simulink model "DC_Motor_project_TET4120 (1)"  (R2024b)
settings: Solver=ode23tb  StartTime=0.0  StopTime=1.2  MaxStep=10e-6  RelTol=1e-3  EnableMultiTasking=on
values from neighbouring files (symbols this model uses):
  A = 2.5    [Other_model_parameters.m]
  c_w = 0.2    [Other_model_parameters.m]
  g = 9.81    [Other_model_parameters.m]
  i_g = 10    [Other_model_parameters.m]
  J = J_car + J_m + J_g    (= 0.50375)    [Other_model_parameters.m]
  M = 2200    [Other_model_parameters.m]
  mu_r = 0.01    [Other_model_parameters.m]
  r_w = 0.25    [Other_model_parameters.m]
  rho = 1.2    [Other_model_parameters.m]
undefined symbols (not defined in the file or in its folder): DiscIntNeverNeededParam, eea_lib, PI, reg
libraries: spsVoltageMeasurementLib x8, simulink_extras x6, spsCurrentMeasurementLib x4, spsOnDelayLib x2, spsMonostableLib x2, spsControlledCurrentSourceLib x2, spsUniversalBridgeLib x2, spsDCVoltageSourceLib x1, sps_lib x1
(part 2 of 2)

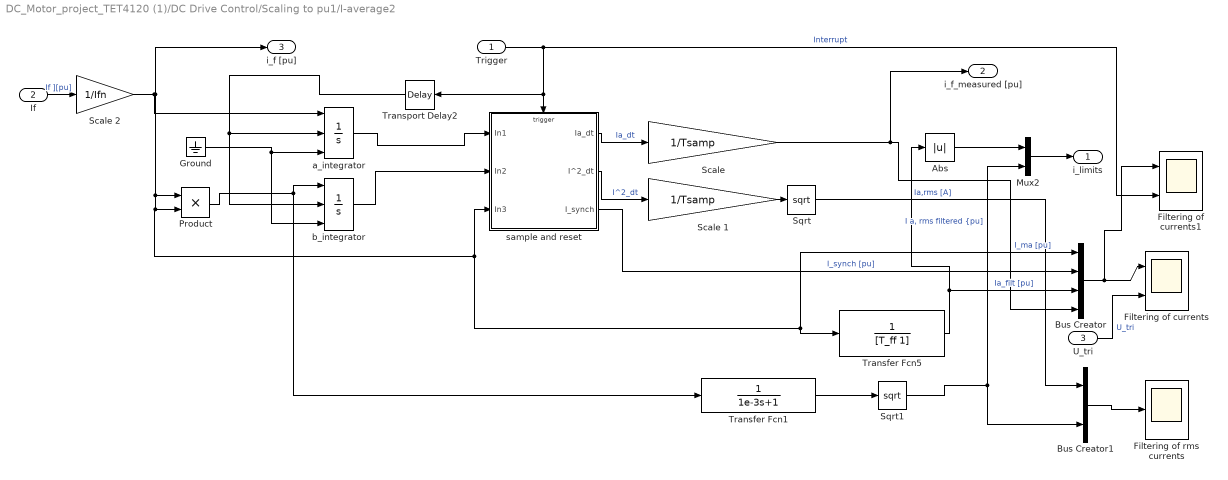
== system DC_Motor_project_TET4120 (1)/DC Drive Control/Scaling to pu1/I-average2 ==
  Trigger : Inport
  If : Inport  Port=2
  U_tri : Inport  Port=3
  Abs : Abs  SaturateOnIntegerOverflow=off
  Bus Creator : BusCreator  Inputs=4
  Bus Creator1 : BusCreator  Inputs=2
  Filtering of currents : Scope  NumInputPorts=2
  Filtering of currents1 : Scope  NumInputPorts=2
  Filtering of rms currents : Scope
  Ground : Ground
  Mux2 : Mux  Inputs=2
  Product : Product  RndMeth=Zero
  "Scale " : Gain  Gain=1/Tsamp
  Scale 1 : Gain  Gain=1/Tsamp
  Scale 2 : Gain  Gain=1/Ifn
  Sqrt : Sqrt
  Sqrt1 : Sqrt
  Transfer Fcn1 : TransferFcn  Denominator=[1e-3 1]
  Transfer Fcn5 : TransferFcn  Denominator=[T_ff 1]
  Transport Delay2 : TransportDelay  DelayTime=1e-12
  a_integrator : Integrator  ExternalReset=rising  InitialConditionSource=external
  b_integrator : Integrator  ExternalReset=rising  InitialConditionSource=external
  sample and reset : Subsystem
  i_limits : Outport
  i_f_measured [pu] : Outport  Port=2
  i_f [pu] : Outport  Port=3
  wires:
  Sqrt/1 -> Bus Creator1/1  "Ia,rms [A]"
  Scale 1/1 -> Sqrt/1
  sample and reset/2(I^2_dt) -> Scale 1/1  "I^2_dt"
  "Scale "/1 -> i_f_measured [pu]/1, Bus Creator/4  "I_ma [pu]"
  sample and reset/1(Ia_dt) -> "Scale "/1  "Ia_dt"
  Product/1 -> b_integrator/1, Transfer Fcn1/1
  Mux2/1 -> i_limits/1
  Transport Delay2/1 -> b_integrator/2, a_integrator/2
  Ground/1 -> b_integrator/3, a_integrator/3
  a_integrator/1 -> sample and reset/1(In1)
  Trigger/1 -> Filtering of currents1/2, Transport Delay2/1, sample and reset/Trigger  "Interrupt"
  Transfer Fcn5/1 -> Bus Creator/3, Abs/1  "Ia_filt [pu]"
  Transfer Fcn1/1 -> Sqrt1/1
  Abs/1 -> Mux2/1
  If/1 -> Scale 2/1  "If ][pu]"
  b_integrator/1 -> sample and reset/2(In2)
  sample and reset/3(I_synch) -> Bus Creator/2  "I_synch [pu]"
  Sqrt1/1 -> Bus Creator1/2, Mux2/2  "I a, rms filtered {pu]"
  Bus Creator/1 -> Filtering of currents1/1, Filtering of currents/1
  Bus Creator1/1 -> Filtering of rms currents/1
  U_tri/1 -> Filtering of currents/2  "U_tri"
  Scale 2/1 -> Bus Creator/1, Transfer Fcn5/1, sample and reset/3(In3), Product/2, Product/1, i_f [pu]/1, a_integrator/1

== system DC_Motor_project_TET4120 (1)/DC Drive Control/Speed Controller/Speed controller  ==
  e : Inport
  UL : Inport  Port=2
  LL : Inport  Port=3
  Abs : Abs  SaturateOnIntegerOverflow=off
  Integral : UnitDelay  SampleTime=-1  HasFrameUpgradeWarning=on
  Kp : Gain  Gain=Kp  SaturateOnIntegerOverflow=on  OutDataTypeStr=Inherit: Same as input  ParamDataTypeStr=Inherit: Same as input
  Lim1 : Subsystem
      mask Display:
      | plot([0.3 0.5 0.7 0.3], [0.1 0.3  0.1 0.1])
      | plot([0.3 0.5 0.7 0.3], [0.9 0.7  0.9 0.9])
  Sum1 : Sum  Inputs=|+-  InputSameDT=on  SaturateOnIntegerOverflow=on  OutDataTypeStr=Inherit: Same as first input
  Sum4 : Sum  Inputs=++|  InputSameDT=on  SaturateOnIntegerOverflow=on  OutDataTypeStr=Inherit: Same as first input
  Switch4 : Switch  Threshold=0.5
  in Limit : Relay  OffSwitchValue=0
  Out : Outport
  wires:
  e/1 -> Kp/1  "e"
  Kp/1 -> Sum4/2
  UL/1 -> Lim1/1(UL)
  Lim1/1(Out) -> Sum1/1, Out/1
  Integral/1 -> Sum4/1, Switch4/1  "intergral"
  Sum4/1 -> Sum1/2, Lim1/2(In), Switch4/3  "u_r"
  LL/1 -> Lim1/3(LL)
  Abs/1 -> in Limit/1
  Sum1/1 -> Abs/1
  in Limit/1 -> Switch4/2  "saturation"
  Switch4/1 -> Integral/1

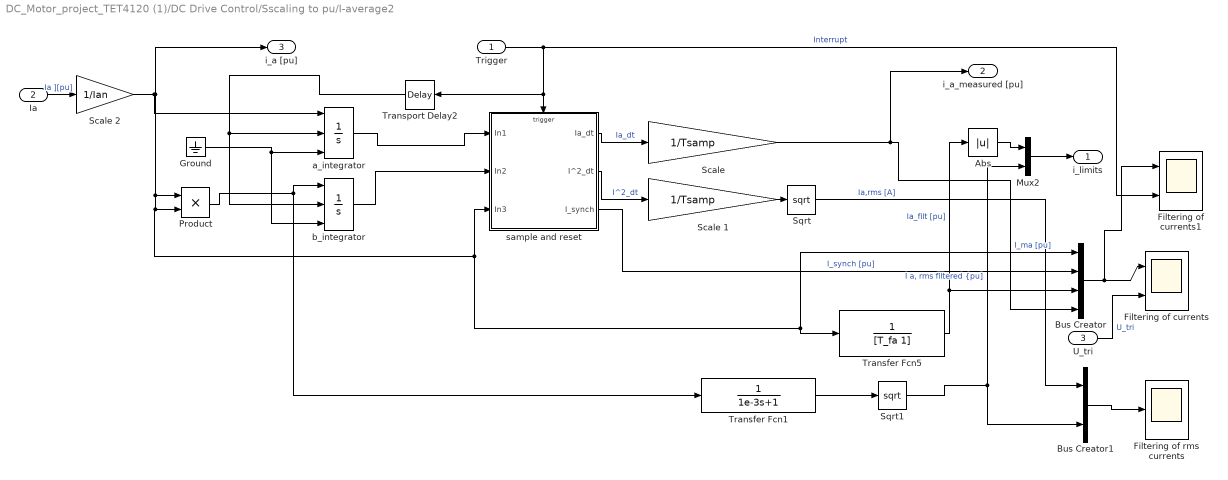
== system DC_Motor_project_TET4120 (1)/DC Drive Control/Sscaling to pu/I-average2 ==
  Trigger : Inport
  Ia : Inport  Port=2
  U_tri : Inport  Port=3
  Abs : Abs  SaturateOnIntegerOverflow=off
  Bus Creator : BusCreator  Inputs=4
  Bus Creator1 : BusCreator  Inputs=2
  Filtering of currents : Scope  NumInputPorts=2
  Filtering of currents1 : Scope  NumInputPorts=2
  Filtering of rms currents : Scope
  Ground : Ground
  Mux2 : Mux  Inputs=2
  Product : Product  RndMeth=Zero
  "Scale " : Gain  Gain=1/Tsamp
  Scale 1 : Gain  Gain=1/Tsamp
  Scale 2 : Gain  Gain=1/Ian
  Sqrt : Sqrt
  Sqrt1 : Sqrt
  Transfer Fcn1 : TransferFcn  Denominator=[1e-3 1]
  Transfer Fcn5 : TransferFcn  Denominator=[T_fa 1]
  Transport Delay2 : TransportDelay  DelayTime=1e-12
  a_integrator : Integrator  ExternalReset=rising  InitialConditionSource=external
  b_integrator : Integrator  ExternalReset=rising  InitialConditionSource=external
  sample and reset : Subsystem
  i_limits : Outport
  i_a_measured [pu] : Outport  Port=2
  i_a [pu] : Outport  Port=3
  wires:
  Sqrt/1 -> Bus Creator1/1  "Ia,rms [A]"
  Scale 1/1 -> Sqrt/1
  sample and reset/2(I^2_dt) -> Scale 1/1  "I^2_dt"
  "Scale "/1 -> i_a_measured [pu]/1, Bus Creator/4  "I_ma [pu]"
  sample and reset/1(Ia_dt) -> "Scale "/1  "Ia_dt"
  Product/1 -> b_integrator/1, Transfer Fcn1/1
  Mux2/1 -> i_limits/1
  Transport Delay2/1 -> b_integrator/2, a_integrator/2
  Ground/1 -> b_integrator/3, a_integrator/3
  a_integrator/1 -> sample and reset/1(In1)
  Trigger/1 -> Filtering of currents1/2, Transport Delay2/1, sample and reset/Trigger  "Interrupt"
  Transfer Fcn5/1 -> Bus Creator/3, Abs/1  "Ia_filt [pu]"
  Transfer Fcn1/1 -> Sqrt1/1
  Abs/1 -> Mux2/1
  Ia/1 -> Scale 2/1  "Ia ][pu]"
  b_integrator/1 -> sample and reset/2(In2)
  sample and reset/3(I_synch) -> Bus Creator/2  "I_synch [pu]"
  Sqrt1/1 -> Bus Creator1/2, Mux2/2  "I a, rms filtered {pu]"
  Bus Creator/1 -> Filtering of currents1/1, Filtering of currents/1
  Bus Creator1/1 -> Filtering of rms currents/1
  U_tri/1 -> Filtering of currents/2  "U_tri"
  Scale 2/1 -> Bus Creator/1, Transfer Fcn5/1, sample and reset/3(In3), Product/2, Product/1, i_a [pu]/1, a_integrator/1

== system DC_Motor_project_TET4120 (1)/DC Drive Control/pwm modulator1/Subsystem ==
  time : Inport
  T_tri : Inport  Port=2
  Abs : Abs
  Bus Creator : BusCreator  Inputs=2
  Constant1 : Constant  Value=4
  Constant2 : Constant
  Gain : Gain  Gain=-1  SaturateOnIntegerOverflow=on  OutDataTypeStr=Inherit: Same as input  ParamDataTypeStr=Inherit: Same as input
  Gain1 : Gain  Gain=-1  SaturateOnIntegerOverflow=on  OutDataTypeStr=Inherit: Same as input  ParamDataTypeStr=Inherit: Same as input
  Product : Product  InputSameDT=on  SaturateOnIntegerOverflow=on  OutDataTypeStr=Inherit: Same as first input
  Product1 : Product  Inputs=*/  InputSameDT=on  SaturateOnIntegerOverflow=on  OutDataTypeStr=Inherit: Same as first input
  Product2 : Product  InputSameDT=on  SaturateOnIntegerOverflow=on  OutDataTypeStr=Inherit: Same as first input
  Product3 : Product  Inputs=*/  InputSameDT=on  SaturateOnIntegerOverflow=on  OutDataTypeStr=Inherit: Same as first input
  Rounding Function : Rounding  Operator=round
  Sum : Sum  Inputs=-+  InputSameDT=on  SaturateOnIntegerOverflow=on  OutDataTypeStr=Inherit: Same as first input
  Sum1 : Sum  Inputs=-+  InputSameDT=on  SaturateOnIntegerOverflow=on  OutDataTypeStr=Inherit: Same as first input
  Out1 : Outport
  wires:
  time/1 -> Sum/1, Product1/1
  T_tri/1 -> Product3/2, Product/2, Product1/2
  Product1/1 -> Rounding Function/1
  Rounding Function/1 -> Product/1
  Product/1 -> Sum/2
  Sum/1 -> Product2/1
  Gain/1 -> Product2/2
  Constant1/1 -> Product3/1
  Product3/1 -> Gain/1
  Product2/1 -> Abs/1
  Abs/1 -> Sum1/2
  Constant2/1 -> Sum1/1
  Gain1/1 -> Bus Creator/1
  Sum1/1 -> Gain1/1, Bus Creator/2
  Bus Creator/1 -> Out1/1

== system DC_Motor_project_TET4120 (1)/DC Drive Control/pwm modulator2/Subsystem ==
  time : Inport
  T_tri : Inport  Port=2
  Abs : Abs
  Bus Creator : BusCreator  Inputs=2
  Constant1 : Constant  Value=4
  Constant2 : Constant
  Gain : Gain  Gain=-1  SaturateOnIntegerOverflow=on  OutDataTypeStr=Inherit: Same as input  ParamDataTypeStr=Inherit: Same as input
  Gain1 : Gain  Gain=-1  SaturateOnIntegerOverflow=on  OutDataTypeStr=Inherit: Same as input  ParamDataTypeStr=Inherit: Same as input
  Product : Product  InputSameDT=on  SaturateOnIntegerOverflow=on  OutDataTypeStr=Inherit: Same as first input
  Product1 : Product  Inputs=*/  InputSameDT=on  SaturateOnIntegerOverflow=on  OutDataTypeStr=Inherit: Same as first input
  Product2 : Product  InputSameDT=on  SaturateOnIntegerOverflow=on  OutDataTypeStr=Inherit: Same as first input
  Product3 : Product  Inputs=*/  InputSameDT=on  SaturateOnIntegerOverflow=on  OutDataTypeStr=Inherit: Same as first input
  Rounding Function : Rounding  Operator=round
  Sum : Sum  Inputs=-+  InputSameDT=on  SaturateOnIntegerOverflow=on  OutDataTypeStr=Inherit: Same as first input
  Sum1 : Sum  Inputs=-+  InputSameDT=on  SaturateOnIntegerOverflow=on  OutDataTypeStr=Inherit: Same as first input
  Out1 : Outport
  wires:
  time/1 -> Sum/1, Product1/1
  T_tri/1 -> Product3/2, Product/2, Product1/2
  Product1/1 -> Rounding Function/1
  Rounding Function/1 -> Product/1
  Product/1 -> Sum/2
  Sum/1 -> Product2/1
  Gain/1 -> Product2/2
  Constant1/1 -> Product3/1
  Product3/1 -> Gain/1
  Product2/1 -> Abs/1
  Abs/1 -> Sum1/2
  Constant2/1 -> Sum1/1
  Gain1/1 -> Bus Creator/1
  Sum1/1 -> Gain1/1, Bus Creator/2
  Bus Creator/1 -> Out1/1

== system DC_Motor_project_TET4120 (1)/DC Drive Control/task manager1/Boolean delay ==
  In1 : Inport
  Data Type Conversion1 : DataTypeConversion  OutDataTypeStr=double  SaturateOnIntegerOverflow=off  RndMeth=Floor
  Data Type Conversion2 : DataTypeConversion  OutDataTypeStr=boolean  SaturateOnIntegerOverflow=off  RndMeth=Floor
  Transport Delay4 : TransportDelay  DelayTime=T_exec_0
  Out1 : Outport
  wires:
  Data Type Conversion2/1 -> Out1/1
  In1/1 -> Data Type Conversion1/1
  Transport Delay4/1 -> Data Type Conversion2/1
  Data Type Conversion1/1 -> Transport Delay4/1

== system DC_Motor_project_TET4120 (1)/DC Drive Control/task manager1/Boolean delay1 ==
  In1 : Inport
  Data Type Conversion1 : DataTypeConversion  OutDataTypeStr=double  SaturateOnIntegerOverflow=off  RndMeth=Floor
  Data Type Conversion2 : DataTypeConversion  OutDataTypeStr=boolean  SaturateOnIntegerOverflow=off  RndMeth=Floor
  Transport Delay4 : TransportDelay  DelayTime=T_exec_0
  Out1 : Outport
  wires:
  Data Type Conversion1/1 -> Transport Delay4/1
  Transport Delay4/1 -> Data Type Conversion2/1
  In1/1 -> Data Type Conversion1/1
  Data Type Conversion2/1 -> Out1/1

== system DC_Motor_project_TET4120 (1)/DC Drive Control/task manager1/Boolean delay2 ==
  In1 : Inport
  Data Type Conversion1 : DataTypeConversion  OutDataTypeStr=double  SaturateOnIntegerOverflow=off  RndMeth=Floor
  Data Type Conversion2 : DataTypeConversion  OutDataTypeStr=boolean  SaturateOnIntegerOverflow=off  RndMeth=Floor
  Transport Delay4 : TransportDelay  DelayTime=T_exec_0
  Out1 : Outport
  wires:
  Data Type Conversion2/1 -> Out1/1
  In1/1 -> Data Type Conversion1/1
  Transport Delay4/1 -> Data Type Conversion2/1
  Data Type Conversion1/1 -> Transport Delay4/1

== system DC_Motor_project_TET4120 (1)/DC Drive Control/task manager1/Int_bottom pulse counter ==
  Trigger : TriggerPort  VariantControl=Variant
  Constant6 : Constant
  Discrete-Time Integrator : DiscreteIntegrator  ExternalReset=level  InitialCondition=1e-3/3  SampleTime=-1  ShowStatePort=on  ICPrevOutput=DiscIntNeverNeededParam  ICPrevScaledInput=DiscIntNeverNeededParam
  Relay1 : Relay  OnSwitchValue=9.3*(1e-3/3)  OffSwitchValue=9.3*(1e-3/3)-eps
  Terminator9 : Terminator
  10th_int_bottom : Outport
  wires:
  Discrete-Time Integrator/1 -> Terminator9/1
  Relay1/1 -> Discrete-Time Integrator/2, 10th_int_bottom/1
  Discrete-Time Integrator/State -> Relay1/1
  Constant6/1 -> Discrete-Time Integrator/1

== system DC_Motor_project_TET4120 (1)/DC Drive Control/Current controller a1/Current controller a/Lim1 ==
  UL : Inport
  In : Inport  Port=2
  LL : Inport  Port=3
  UL test : MinMax  Inputs=2
  UL test1 : MinMax  Function=max  Inputs=2
  Out : Outport
  wires:
  UL test1/1 -> Out/1
  LL/1 -> UL test1/2
  UL test/1 -> UL test1/1
  In/1 -> UL test/2
  UL/1 -> UL test/1

== system DC_Motor_project_TET4120 (1)/DC Drive Control/Current controller a2/Current controller f/Limitation block ==
  UL : Inport
  In : Inport  Port=2
  LL : Inport  Port=3
  UL test : MinMax  Inputs=2
  UL test1 : MinMax  Function=max  Inputs=2
  Out : Outport
  wires:
  UL test1/1 -> Out/1
  LL/1 -> UL test1/2
  UL test/1 -> UL test1/1
  In/1 -> UL test/2
  UL/1 -> UL test/1

== system DC_Motor_project_TET4120 (1)/DC Drive Control/Scaling to pu1/I-average2/sample and reset ==
  In1 : Inport
  In2 : Inport  Port=2
  In3 : Inport  Port=3
  Trigger : TriggerPort  VariantControl=Variant
  Gain : Gain  SaturateOnIntegerOverflow=on  OutDataTypeStr=Inherit: Same as input  ParamDataTypeStr=Inherit: Same as input
  Gain1 : Gain  SaturateOnIntegerOverflow=on  OutDataTypeStr=Inherit: Same as input  ParamDataTypeStr=Inherit: Same as input
  Gain2 : Gain  Gain=0.5
  Gain3 : Gain  Gain=0.5
  Gain4 : Gain  SaturateOnIntegerOverflow=on  OutDataTypeStr=Inherit: Same as input  ParamDataTypeStr=Inherit: Same as input
  Sum : Sum  Inputs=|++
  Sum1 : Sum  Inputs=|++
  Unit Delay : UnitDelay  SampleTime=-1  HasFrameUpgradeWarning=on
  Unit Delay1 : UnitDelay  SampleTime=-1  HasFrameUpgradeWarning=on
  Ia_dt : Outport
  I^2_dt : Outport  Port=2
  I_synch : Outport  Port=3
  wires:
  In2/1 -> Gain1/1
  In1/1 -> Gain/1
  Gain/1 -> Ia_dt/1, Unit Delay/1, Sum/1
  Unit Delay/1 -> Sum/2
  Gain1/1 -> Unit Delay1/1, Sum1/1
  Unit Delay1/1 -> Sum1/2
  Sum/1 -> Gain2/1
  Gain3/1 -> I^2_dt/1
  Sum1/1 -> Gain3/1
  In3/1 -> Gain4/1
  Gain4/1 -> I_synch/1

== system DC_Motor_project_TET4120 (1)/DC Drive Control/Speed Controller/Speed controller /Lim1 ==
  UL : Inport
  In : Inport  Port=2
  LL : Inport  Port=3
  UL test : MinMax  Inputs=2
  UL test1 : MinMax  Function=max  Inputs=2
  Out : Outport
  wires:
  UL test1/1 -> Out/1
  LL/1 -> UL test1/2
  UL test/1 -> UL test1/1
  In/1 -> UL test/2
  UL/1 -> UL test/1

== system DC_Motor_project_TET4120 (1)/DC Drive Control/Sscaling to pu/I-average2/sample and reset ==
  In1 : Inport
  In2 : Inport  Port=2
  In3 : Inport  Port=3
  Trigger : TriggerPort  VariantControl=Variant
  Gain : Gain  SaturateOnIntegerOverflow=on  OutDataTypeStr=Inherit: Same as input  ParamDataTypeStr=Inherit: Same as input
  Gain1 : Gain  SaturateOnIntegerOverflow=on  OutDataTypeStr=Inherit: Same as input  ParamDataTypeStr=Inherit: Same as input
  Gain2 : Gain  Gain=0.5
  Gain3 : Gain  Gain=0.5
  Gain4 : Gain  SaturateOnIntegerOverflow=on  OutDataTypeStr=Inherit: Same as input  ParamDataTypeStr=Inherit: Same as input
  Sum : Sum  Inputs=|++
  Sum1 : Sum  Inputs=|++
  Unit Delay : UnitDelay  SampleTime=-1  HasFrameUpgradeWarning=on
  Unit Delay1 : UnitDelay  SampleTime=-1  HasFrameUpgradeWarning=on
  Ia_dt : Outport
  I^2_dt : Outport  Port=2
  I_synch : Outport  Port=3
  wires:
  In2/1 -> Gain1/1
  In1/1 -> Gain/1
  Gain/1 -> Ia_dt/1, Unit Delay/1, Sum/1
  Unit Delay/1 -> Sum/2
  Gain1/1 -> Unit Delay1/1, Sum1/1
  Unit Delay1/1 -> Sum1/2
  Sum/1 -> Gain2/1
  Gain3/1 -> I^2_dt/1
  Sum1/1 -> Gain3/1
  In3/1 -> Gain4/1
  Gain4/1 -> I_synch/1
